simulink model "mcb_pmsm_foc_hall_hvkit_f28069m"  (R2021b)
settings: Solver=FixedStepDiscrete  StartTime=0.0  StopTime=8  RelTol=1e-3  EnableMultiTasking=on
InitFcn:
  | mcb_pmsm_foc_hall_hvkit_f28069m_data;
values from neighbouring files (symbols this model uses):
  inverter = mcb_SetInverterParameters('BoostXL-DRV8305')    [mcb_pmsm_foc_dual_f28379d_data.m]    (also in mcb_pmsm_foc_dual_f28379d_datascript.m; mcb_pmsm_foc_f280049C_data.m; mcb_pmsm_foc_f28335_data.m = mcb_SetInverterParameters('DRV8312-C2-KIT'); mcb_pmsm_foc_hall_f28035_data.m = mcb_SetInverterParameters('DRV8312-C2-KIT'))
  PI_params = mcb.internal.SetControllerParameters(pmsm,inverter,PU_System,T_pwm,2*Ts,Ts_speed)    [mcb_pmsm_foc_dual_f28379d_data.m]    (also in mcb_pmsm_foc_dual_f28379d_datascript.m; mcb_pmsm_foc_f280049C_data.m = mcb.internal.SetControllerParameters(pmsm,inverter,PU_System; mcb_pmsm_foc_f28335_data.m = mcb.internal.SetControllerParameters(pmsm,inverter,PU_System; mcb_pmsm_foc_hall_f28035_data.m = mcb.internal.SetControllerParameters(pmsm,inverter,PU_System)
  pmsm = struct    [c28335_pmsmfoc_data.m]    (also in mcb_pmsm_foc_dual_f28379d_data.m = mcb_SetPMSMMotorParameters('Teknic2310P'); mcb_pmsm_foc_dual_f28379d_datascript.m = mcb_SetPMSMMotorParameters('Teknic2310P'); mcb_pmsm_foc_f280049C_data.m = mcb_SetPMSMMotorParameters('BLY171D'); mcb_pmsm_foc_f28335_data.m = mcb_SetPMSMMotorParameters('BLY171D'))
  target = mcb_SetProcessorDetails('F28379D',PWM_frequency)    [mcb_pmsm_foc_dual_f28379d_data.m]    (also in mcb_pmsm_foc_dual_f28379d_datascript.m; mcb_pmsm_foc_f280049C_data.m = mcb_SetProcessorDetails('F280049C',PWM_frequency); mcb_pmsm_foc_f28335_data.m = mcb_SetProcessorDetails('F28335',PWM_frequency); mcb_pmsm_foc_hall_f28035_data.m = mcb_SetProcessorDetails('F28035',PWM_frequency))
  Ts = 5e-8    (= 5e-08)    [DCDC_Buck_Param.m]    (also in mcb_c2000_open_loop_control_data.m = T_pwm; mcb_c2000_pmsm_offset_data.m = T_pwm; mcb_pmsm_foc_dual_f28379d_data.m = 5e-05; mcb_pmsm_foc_dual_f28379d_datascript.m = 5e-05)
  Ts_motor = T_pwm/2    (= 2.5e-05)    [mcb_pmsm_foc_dual_f28379d_data.m]    (also in mcb_pmsm_foc_dual_f28379d_datascript.m; mcb_pmsm_foc_f280049C_data.m; mcb_pmsm_foc_f28335_data.m; mcb_pmsm_foc_hall_f28035_data.m)
  Ts_simulink = T_pwm/2    (= 2.5e-05)    [mcb_pmsm_foc_dual_f28379d_data.m]    (also in mcb_pmsm_foc_dual_f28379d_datascript.m; mcb_pmsm_foc_f280049C_data.m; mcb_pmsm_foc_f28335_data.m; mcb_pmsm_foc_hall_f28035_data.m)
undefined symbols (not defined in the file or in its folder): Down, GPTRIP1SEL, GPTRIP2SEL, TZ1, TZ2, Up
libraries: simulink x10, mcbpositiondecoderlib x7, idelinklib_common x5, c2802xlib x5, c280xlib x3, c2806xlib x3, svdutilitieslib x2, mcbcontrolslib x2, demo_controls x1, hall_sensor_lib x1, c2000lib x1, mcbplantlib x1
(part 1 of 2)
settings Model: ExtModeTrigDuration=8  Creator=The MathWorks, Inc.  LastModifiedBy=The MathWorks, Inc.
settings SolverCC: AlgebraicLoopSolver=TrustRegion
settings OptimizationCC: DefaultParameterBehavior=Inlined  DefaultUnderspecifiedDataType=single  OptimizeBlockIOStorage=off  EnhancedBackFolding=on  InitFltsAndDblsToZero=on  NoFixptDivByZeroProtection=on  EfficientFloat2IntCast=on  EfficientMapNaN2IntZero=off  MaxStackSize=1024  OptimizeBlockOrder=speed  DifferentSizesBufferReuse=on  DenormalBehavior=FlushToZero  EfficientTunableParamExpr=on
settings DebuggingCC: ReadBeforeWriteMsg=DisableAll  WriteAfterWriteMsg=DisableAll  WriteAfterReadMsg=DisableAll  InheritedTsInSrcMsg=none  MultiTaskDSMMsg=none  TasksWithSamePriorityMsg=none  IntegerOverflowMsg=none  ParameterPrecisionLossMsg=none  ParameterTunabilityLossMsg=error  SFMachineParentedDataDiag=warning  IntegerSaturationMsg=none
settings HardwareCC: ProdBitPerChar=16  ProdBitPerInt=16  ProdBitPerPointer=32  ProdBitPerSizeT=32  ProdBitPerPtrDiffT=32  ProdLargestAtomicInteger=Integer  ProdLargestAtomicFloat=None  ProdWordSize=16  ProdLongLongMode=on  ProdHWDeviceType=Texas Instruments->C2000
settings SFSimCC: MATLABDynamicMemAlloc=off
settings RTWCC: Description=Embedded Coder  SystemTargetFile=ert.tlc  HardwareBoard=TI Piccolo F2806x  TemplateMakefile=ert_default_tmf  GenerateReport=on  Toolchain=Texas Instruments Code Composer Studio (C2000)
settings CodeAppCC: IgnoreCustomStorageClasses=off  StateflowObjectComments=on
settings ERTTargetCC: CodeReplacementLibrary=TI C28x  ExtModeTransport=3  ExtModeStaticAllocSize=2000  ConvertIfToSwitch=off  SuppressUnreachableDefaultCases=off  MemSecPackage=tic2000demospkg

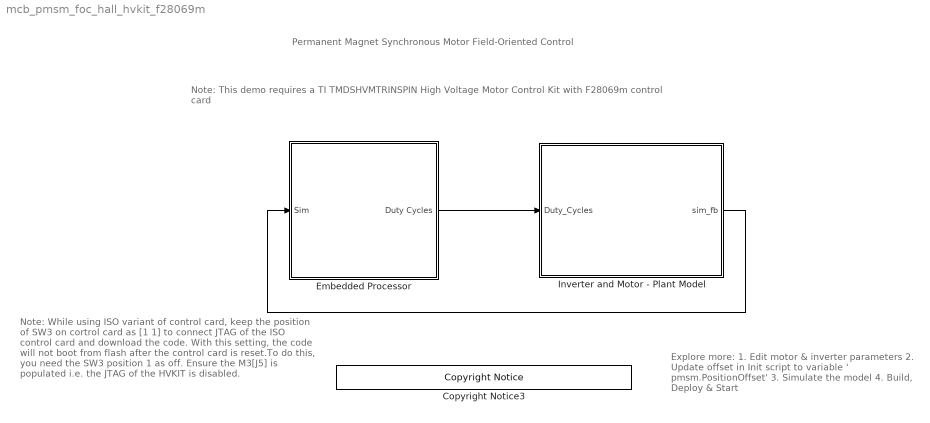
== system mcb_pmsm_foc_hall_hvkit_f28069m ==
  note: Explore more:
      | 1. Edit motor & inverter parameters
      | 2. Update offset in Init script to variable ' pmsm.PositionOffset'
      | 3. Simulate the model
      | 4. Build, Deploy & Start
  note: Permanent Magnet Synchronous Motor Field-Oriented Control
  note: Note: This demo requires a TI TMDSHVMTRINSPIN High Voltage Motor Control Kit with F28069m control card
  note: Note:
      | While using ISO variant of control card, keep the position of SW3 on cortrol card as [1 1] to connect JTAG of the ISO control card and download the code.
      | With this setting, the code will not boot from flash after the control card is reset.To do this, you need the SW3 position 1 as off.
      | Ensure the M3[J5] is populated i.e. the JTAG of the HVKIT is disabled.
  Copyright Notice3 : demo_controls/Copyright Notice  year=2021  prod=tic2000
      settings: SourceProductBaseCode=ME
  Embedded Processor : Subsystem
      mask Display: image('mcb_pmsmfoc_processor.png')
  Inverter and Motor - Plant Model : Subsystem
      mask Display: image('mcb_pmsmfoc_motor.png')
  wires:
  Inverter and Motor - Plant Model/1(sim_fb) -> Embedded Processor/1(Sim)
  Embedded Processor/1(Duty Cycles) -> Inverter and Motor - Plant Model/1(Duty_Cycles)

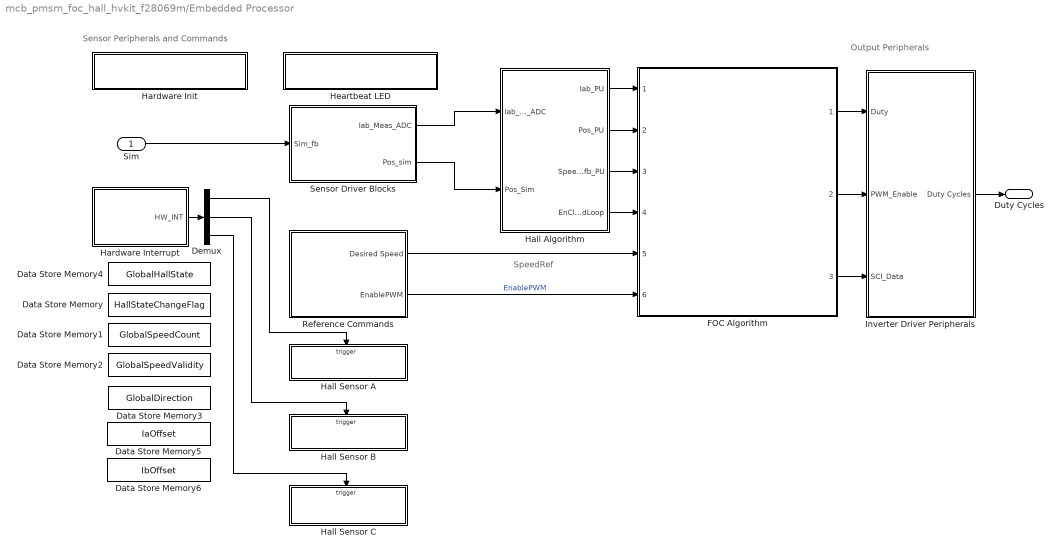
== system mcb_pmsm_foc_hall_hvkit_f28069m/Embedded Processor ==
  note: SpeedRef
  note: Output Peripherals
  note: Sensor Peripherals and Commands
  Sim : Inport
  Data Store Memory : DataStoreMemory  DataStoreName=HallStateChangeFlag  ShowAdditionalParam=off
  Data Store Memory1 : DataStoreMemory  DataStoreName=GlobalSpeedCount  ShowAdditionalParam=off
  Data Store Memory2 : DataStoreMemory  DataStoreName=GlobalSpeedValidity  ShowAdditionalParam=off
  Data Store Memory3 : DataStoreMemory  DataStoreName=GlobalDirection  InitialValue=1  ShowAdditionalParam=off
  Data Store Memory4 : DataStoreMemory  DataStoreName=GlobalHallState  ShowAdditionalParam=off  OutDataTypeStr=uint32
  Data Store Memory5 : DataStoreMemory  DataStoreName=IaOffset  InitialValue=inverter.CtSensAOffset  ShowAdditionalParam=off
  Data Store Memory6 : DataStoreMemory  DataStoreName=IbOffset  InitialValue=inverter.CtSensBOffset  ShowAdditionalParam=off
  Demux : Demux  Outputs=3
  FOC Algorithm : Subsystem  ReferencedSubsystem=foc_hall_algorithm
  Hall Algorithm : Subsystem  TreatAsAtomicUnit=on
      settings: RTWSystemCode=Nonreusable function
  Hall Sensor A : Subsystem
  Hall Sensor B : Subsystem
  Hall Sensor C : Subsystem
  Hardware Init : Subsystem  TreatAsAtomicUnit=on
  Hardware Interrupt : Subsystem  Variant=on  VariantControlMode=sim codegen switching  VariantControl=Choice
  Heartbeat LED : Subsystem  TreatAsAtomicUnit=on
  Inverter Driver Peripherals : Subsystem  TreatAsAtomicUnit=on
      settings: RTWSystemCode=Nonreusable function
  Reference Commands : Subsystem  SystemSampleTime=1e-3
  Sensor Driver Blocks : Subsystem  Variant=on  VariantControlMode=sim codegen switching
  Duty Cycles : Outport
  wires:
  FOC Algorithm/2 -> Inverter Driver Peripherals/2(PWM_Enable)
  Sim/1 -> Sensor Driver Blocks/1(Sim_fb)
  Reference Commands/1(Desired Speed) -> FOC Algorithm/5
  FOC Algorithm/1 -> Inverter Driver Peripherals/1(Duty)
  Inverter Driver Peripherals/1(Duty Cycles) -> Duty Cycles/1
  Reference Commands/2(EnablePWM) -> FOC Algorithm/6  "EnablePWM"
  FOC Algorithm/3 -> Inverter Driver Peripherals/3(SCI_Data)
  Hardware Interrupt/1(HW_INT) -> Demux/1
  Sensor Driver Blocks/1(Iab_Meas_ADC) -> Hall Algorithm/1(Iab_meas_ADC)
  Sensor Driver Blocks/2(Pos_sim) -> Hall Algorithm/2(Pos_Sim)
  Hall Algorithm/1(Iab_PU) -> FOC Algorithm/1
  Hall Algorithm/2(Pos_PU) -> FOC Algorithm/2
  Hall Algorithm/3(Speed_fb_PU) -> FOC Algorithm/3
  Hall Algorithm/4(EnClosedLoop) -> FOC Algorithm/4
  Demux/1 -> Hall Sensor A/Trigger
  Demux/2 -> Hall Sensor B/Trigger
  Demux/3 -> Hall Sensor C/Trigger

== system mcb_pmsm_foc_hall_hvkit_f28069m/Inverter and Motor - Plant Model ==
  Duty_Cycles : Inport
  Bus Creator : BusCreator  Inputs=2
  Plant Model : Subsystem  Variant=on  VariantControlMode=sim codegen switching  VariantControl=Choice
  RT3 : RateTransition  Deterministic=off
  RT4 : RateTransition  Deterministic=off  OutPortSampleTime=Ts
  sim_fb : Outport  VectorParamsAs1DForOutWhenUnconnected=off
  wires:
  Duty_Cycles/1 -> RT3/1
  RT3/1 -> Plant Model/1(Duty_Cycles)
  Plant Model/1(Iab_sim) -> Bus Creator/1  "Iab_sim"
  Plant Model/2(pos_Sim) -> Bus Creator/2  "pos_sim"
  Bus Creator/1 -> RT4/1
  RT4/1 -> sim_fb/1

== system mcb_pmsm_foc_hall_hvkit_f28069m/Embedded Processor/Hall Algorithm ==
  Iab_meas_ADC : Inport
  Pos_Sim : Inport  Port=2
  Input Scaling : Subsystem  Variant=on  VariantControlMode=sim codegen switching  VariantControl=Variant1  PropagateVariantConditions=on
  Iab_PU : Outport
  Pos_PU : Outport  Port=2
  Speed_fb_PU : Outport  Port=3
  EnClosedLoop : Outport  Port=4
  wires:
  Input Scaling/3(Speed_PU) -> Speed_fb_PU/1  "Speed_fb_PU"
  Iab_meas_ADC/1 -> Input Scaling/1(Iab_meas_ADC)
  Input Scaling/4(EnClosedLoop) -> EnClosedLoop/1
  Input Scaling/2(Pos_PU) -> Pos_PU/1  "Pos_PU"
  Pos_Sim/1 -> Input Scaling/2(Pos_Sim)
  Input Scaling/1(Iab_Meas_PU) -> Iab_PU/1  "Iab_PU"

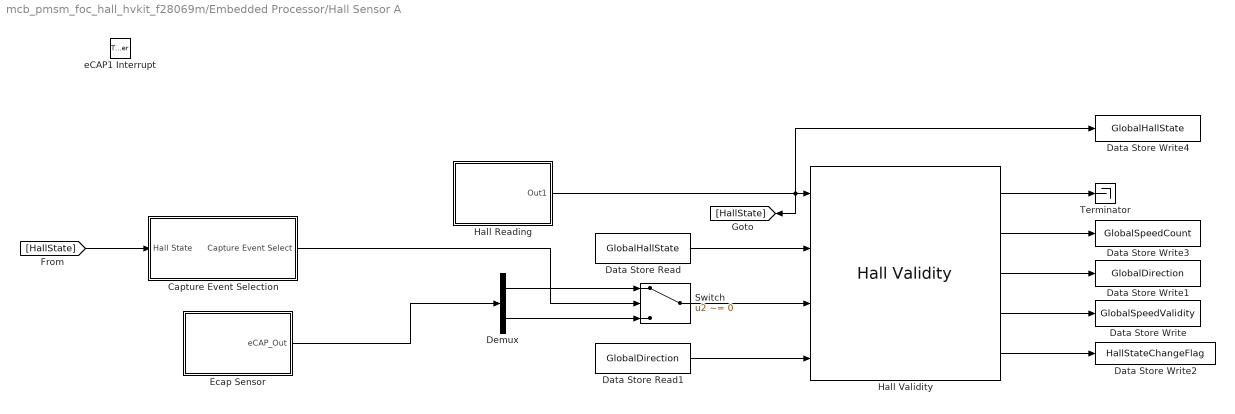
== system mcb_pmsm_foc_hall_hvkit_f28069m/Embedded Processor/Hall Sensor A ==
  eCAP1 Interrupt : TriggerPort  TriggerType=function-call  VariantControl=Variant
  Capture Event Selection : Subsystem
  Data Store Read : DataStoreRead  Priority=1  DataStoreName=GlobalHallState  IndexOptions=Index vector (dialog)  Indices=1  OutputSizes=1
  Data Store Read1 : DataStoreRead  DataStoreName=GlobalDirection  IndexOptions=Index vector (dialog)  Indices=1  OutputSizes=1
  Data Store Write : DataStoreWrite  DataStoreName=GlobalSpeedValidity  IndexOptions=Index vector (dialog)  Indices=1  OutputSizes=1
  Data Store Write1 : DataStoreWrite  DataStoreName=GlobalDirection  IndexOptions=Index vector (dialog)  Indices=1  OutputSizes=1
  Data Store Write2 : DataStoreWrite  DataStoreName=HallStateChangeFlag  IndexOptions=Index vector (dialog)  Indices=1  OutputSizes=1
  Data Store Write3 : DataStoreWrite  DataStoreName=GlobalSpeedCount  IndexOptions=Index vector (dialog)  Indices=1  OutputSizes=1
  Data Store Write4 : DataStoreWrite  Priority=2  DataStoreName=GlobalHallState  IndexOptions=Index vector (dialog)  Indices=1  OutputSizes=1
  Demux : Demux  Outputs=2
  Ecap Sensor : Subsystem  Variant=on  VariantControlMode=sim codegen switching  VariantControl=Choice
  Hall Reading : Subsystem  Variant=on  VariantControlMode=sim codegen switching  VariantControl=Choice
  Hall Validity : mcbpositiondecoderlib/Hall Validity  hallSequence=ABC  sequence=[5,4,6,2,3,1]  CounterSize=32 bits
      settings: SourceProductBaseCode=MT
  Switch : Switch  Criteria=u2 ~= 0
  Terminator : Terminator
  wires:
  Hall Validity/3 -> Data Store Write1/1
  Hall Validity/5 -> Data Store Write2/1
  Hall Validity/4 -> Data Store Write/1
  Data Store Read/1 -> Hall Validity/2
  Data Store Read1/1 -> Hall Validity/4
  Switch/1 -> Hall Validity/3
  Hall Validity/2 -> Data Store Write3/1
  Demux/2 -> Switch/3
  Demux/1 -> Switch/1
  Hall Validity/1 -> Terminator/1
  [HallState] -> Capture Event Selection/1(Hall State)
  Ecap Sensor/1(eCAP_Out) -> Demux/1
  Hall Reading/1(Out1) -> Data Store Write4/1, [HallState], Hall Validity/1
  Capture Event Selection/1(Capture Event Select) -> Switch/2

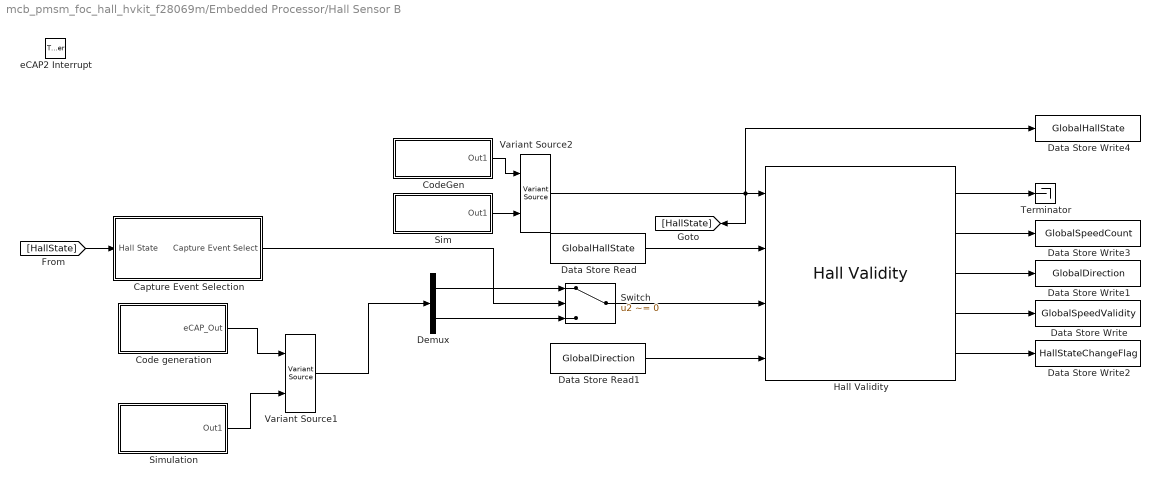
== system mcb_pmsm_foc_hall_hvkit_f28069m/Embedded Processor/Hall Sensor B ==
  eCAP2 Interrupt : TriggerPort  TriggerType=function-call  VariantControl=Variant
  Capture Event Selection : Subsystem
  Code generation : Subsystem
  CodeGen : Subsystem
  Data Store Read : DataStoreRead  Priority=1  DataStoreName=GlobalHallState  IndexOptions=Index vector (dialog)  Indices=1  OutputSizes=1
  Data Store Read1 : DataStoreRead  DataStoreName=GlobalDirection  IndexOptions=Index vector (dialog)  Indices=1  OutputSizes=1
  Data Store Write : DataStoreWrite  DataStoreName=GlobalSpeedValidity  IndexOptions=Index vector (dialog)  Indices=1  OutputSizes=1
  Data Store Write1 : DataStoreWrite  DataStoreName=GlobalDirection  IndexOptions=Index vector (dialog)  Indices=1  OutputSizes=1
  Data Store Write2 : DataStoreWrite  DataStoreName=HallStateChangeFlag  IndexOptions=Index vector (dialog)  Indices=1  OutputSizes=1
  Data Store Write3 : DataStoreWrite  DataStoreName=GlobalSpeedCount  IndexOptions=Index vector (dialog)  Indices=1  OutputSizes=1
  Data Store Write4 : DataStoreWrite  Priority=2  DataStoreName=GlobalHallState  IndexOptions=Index vector (dialog)  Indices=1  OutputSizes=1
  Demux : Demux  Outputs=2
  Hall Validity : mcbpositiondecoderlib/Hall Validity  hallSequence=ABC  sequence=[5,4,6,2,3,1]  CounterSize=32 bits
      settings: SourceProductBaseCode=MT
  Sim : Subsystem
  Simulation : Subsystem
  Switch : Switch  Criteria=u2 ~= 0  Threshold=3
  Terminator : Terminator
  Variant Source1 : VariantSource  VariantControlMode=sim codegen switching
  Variant Source2 : VariantSource  VariantControlMode=sim codegen switching
  wires:
  Hall Validity/3 -> Data Store Write1/1
  Hall Validity/5 -> Data Store Write2/1
  Hall Validity/4 -> Data Store Write/1
  Data Store Read1/1 -> Hall Validity/4
  Hall Validity/2 -> Data Store Write3/1
  Data Store Read/1 -> Hall Validity/2
  Demux/1 -> Switch/1
  Demux/2 -> Switch/3
  Variant Source1/1 -> Demux/1
  Switch/1 -> Hall Validity/3
  Hall Validity/1 -> Terminator/1
  [HallState] -> Capture Event Selection/1(Hall State)
  Capture Event Selection/1(Capture Event Select) -> Switch/2
  Code generation/1(eCAP_Out) -> Variant Source1/1
  Simulation/1(Out1) -> Variant Source1/2
  Variant Source2/1 -> Data Store Write4/1, Hall Validity/1, [HallState]
  CodeGen/1(Out1) -> Variant Source2/1
  Sim/1(Out1) -> Variant Source2/2

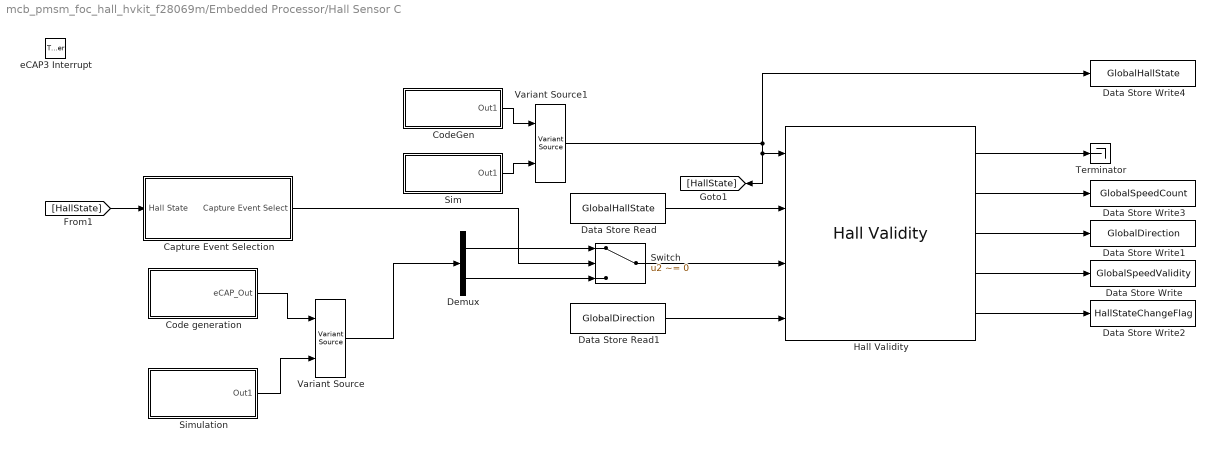
== system mcb_pmsm_foc_hall_hvkit_f28069m/Embedded Processor/Hall Sensor C ==
  eCAP3 Interrupt : TriggerPort  TriggerType=function-call  VariantControl=Variant
  Capture Event Selection : Subsystem
  Code generation : Subsystem
  CodeGen : Subsystem
  Data Store Read : DataStoreRead  Priority=1  DataStoreName=GlobalHallState  IndexOptions=Index vector (dialog)  Indices=1  OutputSizes=1
  Data Store Read1 : DataStoreRead  DataStoreName=GlobalDirection  IndexOptions=Index vector (dialog)  Indices=1  OutputSizes=1
  Data Store Write : DataStoreWrite  DataStoreName=GlobalSpeedValidity  IndexOptions=Index vector (dialog)  Indices=1  OutputSizes=1
  Data Store Write1 : DataStoreWrite  DataStoreName=GlobalDirection  IndexOptions=Index vector (dialog)  Indices=1  OutputSizes=1
  Data Store Write2 : DataStoreWrite  DataStoreName=HallStateChangeFlag  IndexOptions=Index vector (dialog)  Indices=1  OutputSizes=1
  Data Store Write3 : DataStoreWrite  DataStoreName=GlobalSpeedCount  IndexOptions=Index vector (dialog)  Indices=1  OutputSizes=1
  Data Store Write4 : DataStoreWrite  Priority=2  DataStoreName=GlobalHallState  IndexOptions=Index vector (dialog)  Indices=1  OutputSizes=1
  Demux : Demux  Outputs=2
  Hall Validity : mcbpositiondecoderlib/Hall Validity  hallSequence=ABC  sequence=[5,4,6,2,3,1]  CounterSize=32 bits
      settings: SourceProductBaseCode=MT
  Sim : Subsystem
  Simulation : Subsystem
  Switch : Switch  Criteria=u2 ~= 0  Threshold=3
  Terminator : Terminator
  Variant Source : VariantSource  VariantControlMode=sim codegen switching
  Variant Source1 : VariantSource  VariantControlMode=sim codegen switching
  wires:
  Hall Validity/3 -> Data Store Write1/1
  Hall Validity/5 -> Data Store Write2/1
  Hall Validity/4 -> Data Store Write/1
  Data Store Read1/1 -> Hall Validity/4
  Hall Validity/2 -> Data Store Write3/1
  Data Store Read/1 -> Hall Validity/2
  Demux/1 -> Switch/1
  Demux/2 -> Switch/3
  Variant Source/1 -> Demux/1
  Switch/1 -> Hall Validity/3
  Hall Validity/1 -> Terminator/1
  [HallState] -> Capture Event Selection/1(Hall State)
  Capture Event Selection/1(Capture Event Select) -> Switch/2
  Code generation/1(eCAP_Out) -> Variant Source/1
  Simulation/1(Out1) -> Variant Source/2
  Variant Source1/1 -> [HallState], Hall Validity/1, Data Store Write4/1
  CodeGen/1(Out1) -> Variant Source1/1
  Sim/1(Out1) -> Variant Source1/2

== system mcb_pmsm_foc_hall_hvkit_f28069m/Embedded Processor/Hardware Init ==
  Event Listener : EventListener  DisableCoverage=on  EventName=reset
  Offset Calculation : Subsystem  Variant=on  VariantControlMode=sim codegen switching  VariantControl=Choice

== system mcb_pmsm_foc_hall_hvkit_f28069m/Embedded Processor/Hardware Interrupt ==
  Code Generation : Subsystem  VariantControl=(codegen)
  Simulation : Subsystem  VariantControl=(sim)
  HW_INT : Outport  OutputFunctionCall=on

== system mcb_pmsm_foc_hall_hvkit_f28069m/Embedded Processor/Heartbeat LED ==
  note: Heartbeat LED 1HZ
  LED BLINK : Subsystem  Variant=on  VariantControlMode=sim codegen switching  VariantControl=Choice
  RED_LED : Constant  OutDataTypeStr=uint16  SampleTime=0.5
  wires:
  RED_LED/1 -> LED BLINK/1(In1)

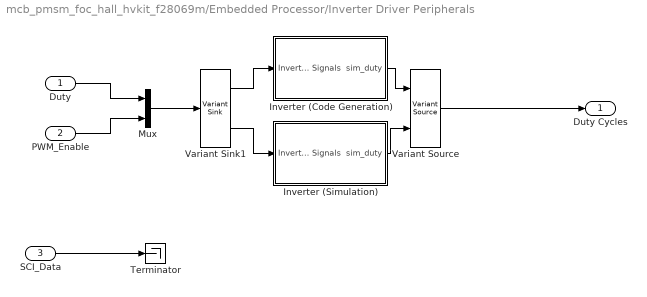
== system mcb_pmsm_foc_hall_hvkit_f28069m/Embedded Processor/Inverter Driver Peripherals ==
  Duty : Inport
  PWM_Enable : Inport  Port=2
  SCI_Data : Inport  Port=3
  Inverter (Code Generation) : Subsystem  VariantControl=Choice
  Inverter (Simulation) : Subsystem  VariantControl=(sim)
  Mux : Mux  Inputs=2
  Terminator : Terminator
  Variant Sink1 : VariantSink  VariantControlMode=sim codegen switching
  Variant Source : VariantSource  VariantControlMode=sim codegen switching
  Duty Cycles : Outport  InitialOutput=0  VectorParamsAs1DForOutWhenUnconnected=off
  wires:
  Variant Source/1 -> Duty Cycles/1
  PWM_Enable/1 -> Mux/2
  Duty/1 -> Mux/1
  Variant Sink1/2 -> Inverter (Simulation)/1(Inverter Signals)
  Inverter (Code Generation)/1(sim_duty) -> Variant Source/1
  Mux/1 -> Variant Sink1/1
  Variant Sink1/1 -> Inverter (Code Generation)/1(Inverter Signals)
  Inverter (Simulation)/1(sim_duty) -> Variant Source/2
  SCI_Data/1 -> Terminator/1

== system mcb_pmsm_foc_hall_hvkit_f28069m/Embedded Processor/Reference Commands ==
  Data Type Conversion3 : DataTypeConversion  OutDataTypeStr=boolean  RndMeth=Simplest
  Enable PWM : Constant  OutDataTypeStr=uint16
  Speed Command in PU : Constant  Value=0.5  OutDataTypeStr=dataType
  Desired Speed : Outport  VectorParamsAs1DForOutWhenUnconnected=off
  EnablePWM : Outport  Port=2
  wires:
  Data Type Conversion3/1 -> EnablePWM/1
  Speed Command in PU/1 -> Desired Speed/1  "Speed_Ref"
  Enable PWM/1 -> Data Type Conversion3/1

== system mcb_pmsm_foc_hall_hvkit_f28069m/Embedded Processor/Sensor Driver Blocks ==
  Sim_fb : Inport
  Sensor Driver Blocks (codegen) : Subsystem  VariantControl=(codegen)
  Sensor Driver Blocks (sim) : Subsystem  VariantControl=(sim)
  Iab_Meas_ADC : Outport
  Pos_sim : Outport  Port=2

== system mcb_pmsm_foc_hall_hvkit_f28069m/Inverter and Motor - Plant Model/Plant Model ==
  Duty_Cycles : Inport
  Codegeneration : Subsystem  VariantControl=(codegen)
  Simulation : Subsystem  VariantControl=(sim)
  Iab_sim : Outport
  pos_Sim : Outport  Port=2

== system mcb_pmsm_foc_hall_hvkit_f28069m/Embedded Processor/Hall Algorithm/Input Scaling ==
  note: Variant control to pass plant simulated value for simulation and
      | ADC measured value for codegen.
  Iab_meas_ADC : Inport
  Pos_Sim : Inport  Port=2
  Read_Sensor (codegen) : Subsystem  VariantControl=(codegen)
  Read_Sensor (sim) : Subsystem  VariantControl=(sim)
  Iab_Meas_PU : Outport  VectorParamsAs1DForOutWhenUnconnected=off
  Pos_PU : Outport  Port=2  VectorParamsAs1DForOutWhenUnconnected=off
  Speed_PU : Outport  Port=3  VectorParamsAs1DForOutWhenUnconnected=off
  EnClosedLoop : Outport  Port=4  VectorParamsAs1DForOutWhenUnconnected=off

== system mcb_pmsm_foc_hall_hvkit_f28069m/Embedded Processor/Hall Sensor A/Capture Event Selection ==
  Hall State : Inport
  If : If  IfExpression=(u1 == 5 | u1 == 3)
  Merge : Merge
  Output 0 : Subsystem  TreatAsAtomicUnit=on
  Output 1 : Subsystem  TreatAsAtomicUnit=on
  Capture Event Select : Outport
  wires:
  Output 1/1(Out1) -> Merge/2
  Output 0/1(Out1) -> Merge/1
  If/2 -> Output 1/Action
  If/1 -> Output 0/Action
  Hall State/1 -> If/1
  Merge/1 -> Capture Event Select/1

== system mcb_pmsm_foc_hall_hvkit_f28069m/Embedded Processor/Hall Sensor A/Ecap Sensor ==
  Code generation : Subsystem  VariantControl=(codegen)
  Simulation : Subsystem  VariantControl=(sim)
  eCAP_Out : Outport

== system mcb_pmsm_foc_hall_hvkit_f28069m/Embedded Processor/Hall Sensor A/Hall Reading ==
  CodeGen : Subsystem  VariantControl=(codegen)
  Sim : Subsystem  VariantControl=(sim)
  Out1 : Outport

== system mcb_pmsm_foc_hall_hvkit_f28069m/Embedded Processor/Hall Sensor B/Capture Event Selection ==
  Hall State : Inport
  If : If  IfExpression=(u1 == 3 | u1 == 6)
  Merge : Merge
  Output 0 : Subsystem  TreatAsAtomicUnit=on
  Output 1 : Subsystem  TreatAsAtomicUnit=on
  Capture Event Select : Outport
  wires:
  Output 1/1(Out1) -> Merge/1
  Output 0/1(Out1) -> Merge/2
  If/2 -> Output 0/Action
  If/1 -> Output 1/Action
  Hall State/1 -> If/1
  Merge/1 -> Capture Event Select/1

== system mcb_pmsm_foc_hall_hvkit_f28069m/Embedded Processor/Hall Sensor B/Code generation ==
  eCAP : c280xlib/eCAP  operatingMode=eCAP  selectCAPx=eCAP2  offsetValue=0  counterSynIn=off  enableCounter=off  syncOutput=Disabled  sampleTime=-1  eventPrescaler=0  selectMode=Continuous  enableOneShot=off  stopValue=Capture Event 2  resetEv1Ts=on  ev1Polarity=Rising Edge  resetEv2Ts=on  ev2Polarity=Falling Edge  resetEv3Ts=off  ev3Polarity=Rising Edge  resetEv4Ts=off  ev4Polarity=Rising Edge  tSCntrDataType=uint32  capEvFlag=off  capFlagDataType=uint16  overFlowFlag=off  overFlowFlagDataType=uint16  periodUnit=Seconds  periodSource=Specify via dialog  waveformPeriod=0.001  dutyUnit=Percentages  dutySource=Specify via dialog  dutyCycle=50  outputPolarity=Active High  enableCEVT1Int=on  enableCEVT2Int=on  enableCEVT3Int=off  enableCEVT4Int=off  enableCTROVFInt=on  enablePRDInt=off  enableCMPInt=off
      settings: SourceProductBaseCode=TIC2000
  eCAP_Out : Outport
  wires:
  eCAP/1 -> eCAP_Out/1

== system mcb_pmsm_foc_hall_hvkit_f28069m/Embedded Processor/Hall Sensor B/CodeGen ==
  Bitwise AND : simulink/Logic and Bit Operations/Bitwise Operator  logicop=AND  UseBitMask=on  BitMask=hex2dec('07000000')  BitMaskRealWorld=Stored Integer
  Data Type Conversion : DataTypeConversion  OutDataTypeStr=uint32  ConvertRealWorld=Stored Integer (SI)
  Memory Copy : idelinklib_common/Memory Copy  copyFrom=Specified source code symbol  copyFromAddressSource=Specify via dialog  copyFromAddress=hex2dec('00001000')  copyFromSrcCode=&GpioDataRegs.GPADAT.all  dataTypeFrom=uint32  dataDimensionFrom=1  useOffsetFrom=off  offsetFromSrc=Specify via dialog  offsetFrom=0  strideFrom=1  copyTo=Output port  copyToAddressSource=Specify via dialog  copyToAddress=hex2dec('00002000')  copyToSrcCode=myVariableDst  dataTypeTo=uint32  useOffsetTo=off  offsetToSrc=Specify via dialog  offsetTo=0  strideTo=1  sampleTime=-1  useInitValue=off  initValueSrc=Specify constant value  initValue=1  initValueSrcCode=myInitValueVariable  useAsMask=off  maskOperator=bitwise AND  useTermValue=off  termValue=1  isRealtimeEnabled=off  emitCCBeforeWrite=off  CCBeforeWrite=/* Custom Code Before Write*/  emitCCAfterWrite=off  CCAfterWrite=/* Custom Code After Write*/  useDMACopy=off  enableBlockingMode=off
      settings: SourceProductBaseCode=ME
  Shift Arithmetic : ArithShift  BitShiftNumber=24
  Out1 : Outport
  wires:
  Memory Copy/1 -> Bitwise AND/1
  Data Type Conversion/1 -> Out1/1
  Bitwise AND/1 -> Shift Arithmetic/1
  Shift Arithmetic/1 -> Data Type Conversion/1

== system mcb_pmsm_foc_hall_hvkit_f28069m/Embedded Processor/Hall Sensor B/Sim ==
  Data Type Conversion : DataTypeConversion  OutDataTypeStr=uint32  ConvertRealWorld=Stored Integer (SI)
  Ground : Ground
  Out1 : Outport
  wires:
  Data Type Conversion/1 -> Out1/1
  Ground/1 -> Data Type Conversion/1

== system mcb_pmsm_foc_hall_hvkit_f28069m/Embedded Processor/Hall Sensor B/Simulation ==
  Ground : Ground
  Ground1 : Ground
  Mux : Mux  Inputs=2
  Out1 : Outport
  wires:
  Ground1/1 -> Mux/2
  Mux/1 -> Out1/1
  Ground/1 -> Mux/1

== system mcb_pmsm_foc_hall_hvkit_f28069m/Embedded Processor/Hall Sensor C/Capture Event Selection ==
  Hall State : Inport
  If : If  IfExpression=(u1 == 5 | u1 == 6)
  Merge : Merge
  Output 0 : Subsystem  TreatAsAtomicUnit=on
  Output 1 : Subsystem  TreatAsAtomicUnit=on
  Capture Event Select : Outport
  wires:
  Output 1/1(Out1) -> Merge/1
  Output 0/1(Out1) -> Merge/2
  If/2 -> Output 0/Action
  If/1 -> Output 1/Action
  Hall State/1 -> If/1
  Merge/1 -> Capture Event Select/1

== system mcb_pmsm_foc_hall_hvkit_f28069m/Embedded Processor/Hall Sensor C/Code generation ==
  eCAP : c280xlib/eCAP  operatingMode=eCAP  selectCAPx=eCAP3  offsetValue=0  counterSynIn=off  enableCounter=off  syncOutput=Disabled  sampleTime=-1  eventPrescaler=0  selectMode=Continuous  enableOneShot=off  stopValue=Capture Event 2  resetEv1Ts=on  ev1Polarity=Rising Edge  resetEv2Ts=on  ev2Polarity=Falling Edge  resetEv3Ts=off  ev3Polarity=Rising Edge  resetEv4Ts=off  ev4Polarity=Rising Edge  tSCntrDataType=uint32  capEvFlag=off  capFlagDataType=uint16  overFlowFlag=off  overFlowFlagDataType=uint16  periodUnit=Seconds  periodSource=Specify via dialog  waveformPeriod=0.001  dutyUnit=Percentages  dutySource=Specify via dialog  dutyCycle=50  outputPolarity=Active High  enableCEVT1Int=on  enableCEVT2Int=on  enableCEVT3Int=off  enableCEVT4Int=off  enableCTROVFInt=on  enablePRDInt=off  enableCMPInt=off
      settings: SourceProductBaseCode=TIC2000
  eCAP_Out : Outport
  wires:
  eCAP/1 -> eCAP_Out/1

== system mcb_pmsm_foc_hall_hvkit_f28069m/Embedded Processor/Hall Sensor C/CodeGen ==
  Bitwise AND : simulink/Logic and Bit Operations/Bitwise Operator  logicop=AND  UseBitMask=on  BitMask=hex2dec('07000000')  BitMaskRealWorld=Stored Integer
  Data Type Conversion : DataTypeConversion  OutDataTypeStr=uint32  ConvertRealWorld=Stored Integer (SI)
  Memory Copy : idelinklib_common/Memory Copy  copyFrom=Specified source code symbol  copyFromAddressSource=Specify via dialog  copyFromAddress=hex2dec('00001000')  copyFromSrcCode=&GpioDataRegs.GPADAT.all  dataTypeFrom=uint32  dataDimensionFrom=1  useOffsetFrom=off  offsetFromSrc=Specify via dialog  offsetFrom=0  strideFrom=1  copyTo=Output port  copyToAddressSource=Specify via dialog  copyToAddress=hex2dec('00002000')  copyToSrcCode=myVariableDst  dataTypeTo=uint32  useOffsetTo=off  offsetToSrc=Specify via dialog  offsetTo=0  strideTo=1  sampleTime=-1  useInitValue=off  initValueSrc=Specify constant value  initValue=1  initValueSrcCode=myInitValueVariable  useAsMask=off  maskOperator=bitwise AND  useTermValue=off  termValue=1  isRealtimeEnabled=off  emitCCBeforeWrite=off  CCBeforeWrite=/* Custom Code Before Write*/  emitCCAfterWrite=off  CCAfterWrite=/* Custom Code After Write*/  useDMACopy=off  enableBlockingMode=off
      settings: SourceProductBaseCode=ME
  Shift Arithmetic : ArithShift  BitShiftNumber=24
  Out1 : Outport
  wires:
  Data Type Conversion/1 -> Out1/1
  Shift Arithmetic/1 -> Data Type Conversion/1
  Bitwise AND/1 -> Shift Arithmetic/1
  Memory Copy/1 -> Bitwise AND/1

== system mcb_pmsm_foc_hall_hvkit_f28069m/Embedded Processor/Hall Sensor C/Sim ==
  Data Type Conversion : DataTypeConversion  OutDataTypeStr=uint32  ConvertRealWorld=Stored Integer (SI)
  Ground : Ground
  Out1 : Outport
  wires:
  Data Type Conversion/1 -> Out1/1
  Ground/1 -> Data Type Conversion/1

== system mcb_pmsm_foc_hall_hvkit_f28069m/Embedded Processor/Hall Sensor C/Simulation ==
  Ground : Ground
  Ground1 : Ground
  Mux : Mux  Inputs=2
  Out1 : Outport
  wires:
  Ground1/1 -> Mux/2
  Mux/1 -> Out1/1
  Ground/1 -> Mux/1

== system mcb_pmsm_foc_hall_hvkit_f28069m/Embedded Processor/Hardware Init/Offset Calculation ==
  Code Generation : Subsystem  VariantControl=(codegen)
  Simulation : Subsystem  VariantControl=(sim)

== system mcb_pmsm_foc_hall_hvkit_f28069m/Embedded Processor/Hardware Interrupt/Code Generation ==
  Hardware Interrupt : c2000lib/Scheduling/C28x Hardware Interrupt  irqnumbers=[4 4 4]  pienumbers=[1 2 3]  irqpriorities=[25 25 25]  irqpreempts=[0 0 0]  showinput=off  dspchiptype=C280X
      settings: SourceProductBaseCode=TIC2000
  HW_INT : Outport  VectorParamsAs1DForOutWhenUnconnected=off
  wires:
  Hardware Interrupt/1 -> HW_INT/1

== system mcb_pmsm_foc_hall_hvkit_f28069m/Embedded Processor/Hardware Interrupt/Simulation ==
  Function-Call Generator1 : simulink/Ports & Subsystems/Function-Call Generator  sample_time=Ts  numberOfIterations=1  DisallowWideOutput=off
  Function-Call Generator3 : simulink/Ports & Subsystems/Function-Call Generator  sample_time=Ts  numberOfIterations=1  DisallowWideOutput=off
  Function-Call Generator4 : simulink/Ports & Subsystems/Function-Call Generator  sample_time=Ts  numberOfIterations=1  DisallowWideOutput=off
  Mux : Mux  Inputs=3
  HW_INT : Outport  VectorParamsAs1DForOutWhenUnconnected=off
  wires:
  Mux/1 -> HW_INT/1
  Function-Call Generator1/1 -> Mux/1
  Function-Call Generator3/1 -> Mux/2
  Function-Call Generator4/1 -> Mux/3

== system mcb_pmsm_foc_hall_hvkit_f28069m/Embedded Processor/Heartbeat LED/LED BLINK ==
  In1 : Inport
  Code generation : Subsystem  VariantControl=(codegen)
  Simulation : Subsystem  VariantControl=(sim)

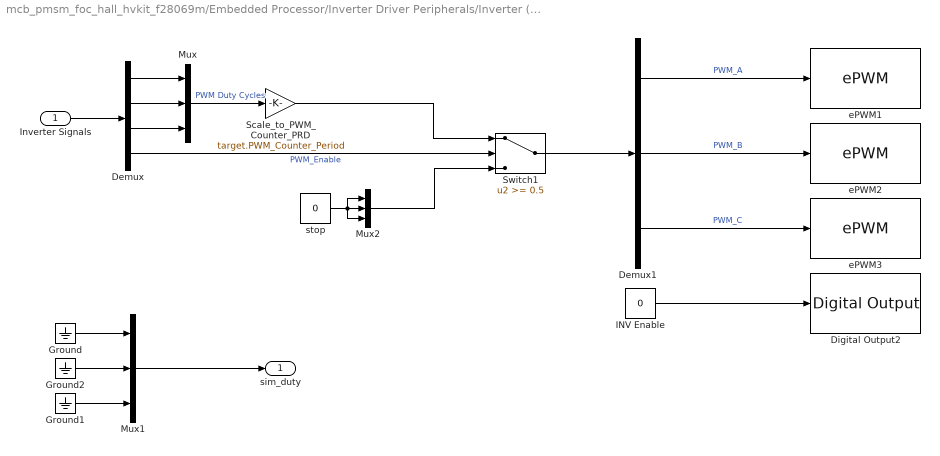
== system mcb_pmsm_foc_hall_hvkit_f28069m/Embedded Processor/Inverter Driver Peripherals/Inverter (Code Generation) ==
  Inverter Signals : Inport
  Demux : Demux
  Demux1 : Demux  Outputs=3
  Digital Output2 : c2806xlib/Digital Output  GPIO_Number=GPIO8~GPIO15  GPIO_Bit0=off  GPIO_BIT0_Toggle=off  GPIO_Bit1=off  GPIO_BIT1_Toggle=off  GPIO_Bit2=off  GPIO_BIT2_Toggle=off  GPIO_Bit3=off  GPIO_BIT3_Toggle=off  GPIO_Bit4=off  GPIO_BIT4_Toggle=off  GPIO_Bit5=off  GPIO_BIT5_Toggle=off  GPIO_Bit6=off  GPIO_BIT6_Toggle=off  GPIO_Bit7=on  GPIO_BIT7_Toggle=off
      settings: SourceProductBaseCode=TIC2000
  Ground : Ground
  Ground1 : Ground
  Ground2 : Ground
  INV Enable : Constant  Value=0  OutDataTypeStr=uint16
  Mux : Mux  Inputs=3
  Mux1 : Mux  Inputs=3
  Mux2 : Mux  Inputs=3
  Scale_to_PWM_Counter_PRD : Gain  Gain=target.PWM_Counter_Period  OutDataTypeStr=uint16  RndMeth=Simplest
  Switch1 : Switch  Threshold=0.5
  ePWM1 : c2802xlib/ePWM  PwmType=C2000  useModule=ePWM1  ePWMxLINKTBPRD=Not Linked  periodUnits=Clock cycles  timerSource=Specify via dialog  timerPeriod_clk=target.PWM_Counter_Period+1  timerPeriod_sec=64000  tbshadow=Counter equals to zero  countingMode=Up-Down  phaseActiveEnable=Disable  phaseDirection=Count down after sync  phaseActive=0  synchronizationEnable=off  dcaevt1Sync=off  dcbevt1Sync=off  synchronizationOption=Counter equals to zero (CTR=Zero)  perSynchronizationOption=Counter equals to period (CTR=PRD)  clockPrescale=1  HSclockPrescale=1  enswap=off  ePWMxAStatus=on  ePWMxAactionLogic1=Do nothing  ePWMxAactionLogic2=Do nothing  ePWMxAactionLogic3=Clear  ePWMxAactionLogic4=Set  ePWMxAactionLogic5=Do nothing  ePWMxAactionLogic6=Do nothing  ePWMxACSFenable=off  ePWMxACSFvalue=Forcing disable  ePWMxASFreload=Zero  ePWMxBStatus=off  ePWMxBactionLogic1=Do nothing  ePWMxBactionLogic2=Set  ePWMxBactionLogic3=Do nothing  ePWMxBactionLogic4=Do nothing  ePWMxBactionLogic5=Clear  ePWMxBactionLogic6=Do nothing  ePWMxBCSFenable=off  ePWMxBCSFvalue=Forcing disable  ePWMxBSFreload=Zero  ePWNxBOutWay=off  ePWMxLINKCMPA=Not Linked  CMPAUnits=Clock cycles  CMPASource=Input port  CMPAValue_per=32000  CMPAValue_clk=target.PWM_Counter_Period/2+1  enCMPAshadow=Counter equals to zero (CTR=Zero)  ePWMxLINKCMPB=Not Linked  CMPBUnits=Clock cycles  CMPBSource=Specify via dialog  CMPBValue_per=50  CMPBValue_clk=target.PWM_Counter_Period/2+1  enCMPBshadow=Counter equals to zero (CTR=Zero)  ePWMxLINKCMPC=Not Linked  CMPCUnits=Clock cycles  CMPCSource=Specify via dialog  CMPCValue_per=50  CMPCValue_clk=32000  enCMPCshadow=Counter equals to zero (CTR=Zero)  ePWMxLINKCMPD=Not Linked  CMPDUnits=Clock cycles  CMPDSource=Specify via dialog  CMPDValue_per=50  CMPDValue_clk=32000  enCMPDshadow=Counter equals to zero (CTR=Zero)  enableDBePWMxA=on  enableDBePWMxB=on  enhalfcycle=off  DBpolarity=Active high complementary (AHC)  DBedgeDelay=Positive  DBSource_ePWMxA=ePWMxA  DBSource_ePWMxB=ePWMxA  DBPeriodUnits=Clock cycles  DBperiodSource=Specify via dialog  REDperiod=15  FEDperiod=15  REDperiod_sec=0  FEDperiod_sec=0  LoadModeDBRED=Immediate without using shadow  LoadModeDBFED=Immediate without using shadow  adcstartModuleA=on  adcrequestEventA=First event  adcstartEventA=Counter equals to period (CTR=PRD)  adcstartEventA_type2=Digital Compare Module A Event 1 start of conversion (DCAEVT1.soc)  adcstartModuleB=off  adcrequestEventB=First event  adcstartEventB=Counter equals to zero (CTR=Zero)  adcstartEventB_type2=Counter equals to zero (CTR=Zero)  intEn=off  intPrd=First event  intSel=Counter equals to zero (CTR=Zero)  intSel_type2=Counter equals to zero (CTR=Zero)  hrpe=off  enHRPWM=off  HRPWM_LoadMode=Counter equals to period (CTR=PRD)  HRPWM_CTLMode=Duty or Period control mode  HRPWM_EDGMode=Both edge  hrpeb=off  enHRPWMB=off  HRPWM_LoadModeB=Counter equals to zero (CTR=ZERO)  HRPWM_CTLModeB=Duty or Period control mode  HRPWM_EDGModeB=Both edge  enHRDBRED=off  enHRDBFED=off  enSFO=on  enautoconv=on  chopperEnable=off  chopperFrequency=1  chopperFirstwidth=1  chopperDuty=12.5%  tripZonesource=Specify via dialog  tzselOSHT1=off  tzselOSHT2=off  tzselOSHT3=off  tzselOSHDCAEV1=off  tzselOSHDCBEV1=off  tzselCBC1=off  tzselCBC2=off  tzselCBC3=off  tzselCBCDCAEV2=off  tzselCBCDCBEV2=off  tzselOSHT4=off  tzselOSHT5=off  tzselOSHT6=off  tzselCBC4=off  tzselCBC5=off  tzselCBC6=off  enTzOstIntr=off  enTzCbcIntr=off  enTzDCAEVT1Intr=off  enTzDCAEVT2Intr=off  enTzDCBEVT1Intr=off  enTzDCBEVT2Intr=off  ePWMxAforced=No action  ePWMxBforced=No action  DCAEVT1forced=No action  DCBEVT1forced=No action  DCAEVT2forced=No action  DCBEVT2forced=No action  dcah=Trip Zone 1 input (TZ1)  dcal=Trip Zone 2 input (TZ2)  dcbh=Trip Zone 1 input (TZ1)  dcbl=Trip Zone 2 input (TZ2)  dcah_type2=GPTRIP1SEL/(TZ1)  dcal_type2=GPTRIP2SEL/(TZ2)  dcbh_type2=GPTRIP1SEL/(TZ1)  dcbl_type2=GPTRIP2SEL/(TZ2)  gendcaevt1=Event disabled  gendcaevt2=Event disabled  gendcbevt1=Event disabled  gendcbevt2=Event disabled  dcaevt1src=DCAEVT1 with sync  dcaevt2src=DCAEVT2 with sync  dcbevt1src=DCBEVT1 with sync  dcbevt2src=DCBEVT2 with sync  pulsesel=Counter equals to zero (CTR=Zero)  blankinv=off  blankoffset=0  blankwidth=0  evsrcsel=Filtered version of DCAEVT1 (DCAEVT1FILT)  encape=off
  ePWM2 : c2802xlib/ePWM  PwmType=C2000  useModule=ePWM2  ePWMxLINKTBPRD=Not Linked  periodUnits=Clock cycles  timerSource=Specify via dialog  timerPeriod_clk=target.PWM_Counter_Period+1  timerPeriod_sec=64000  tbshadow=Counter equals to zero  countingMode=Up-Down  phaseActiveEnable=Set counter to phase value specified via dialog  phaseDirection=Count up after sync  phaseActive=0  synchronizationEnable=off  dcaevt1Sync=off  dcbevt1Sync=off  synchronizationOption=Pass through (EPWMxSYNCI or SWFSYNC)  perSynchronizationOption=Counter equals to period (CTR=PRD)  clockPrescale=1  HSclockPrescale=1  enswap=off  ePWMxAStatus=on  ePWMxAactionLogic1=Do nothing  ePWMxAactionLogic2=Do nothing  ePWMxAactionLogic3=Clear  ePWMxAactionLogic4=Set  ePWMxAactionLogic5=Do nothing  ePWMxAactionLogic6=Do nothing  ePWMxACSFenable=off  ePWMxACSFvalue=Forcing disable  ePWMxASFreload=Zero  ePWMxBStatus=off  ePWMxBactionLogic1=Do nothing  ePWMxBactionLogic2=Set  ePWMxBactionLogic3=Do nothing  ePWMxBactionLogic4=Do nothing  ePWMxBactionLogic5=Clear  ePWMxBactionLogic6=Do nothing  ePWMxBCSFenable=off  ePWMxBCSFvalue=Forcing disable  ePWMxBSFreload=Zero  ePWNxBOutWay=off  ePWMxLINKCMPA=Not Linked  CMPAUnits=Clock cycles  CMPASource=Input port  CMPAValue_per=32000  CMPAValue_clk=target.PWM_Counter_Period/2+1  enCMPAshadow=Counter equals to zero (CTR=Zero)  ePWMxLINKCMPB=Not Linked  CMPBUnits=Clock cycles  CMPBSource=Specify via dialog  CMPBValue_per=50  CMPBValue_clk=target.PWM_Counter_Period/2+1  enCMPBshadow=Counter equals to zero (CTR=Zero)  ePWMxLINKCMPC=Not Linked  CMPCUnits=Clock cycles  CMPCSource=Specify via dialog  CMPCValue_per=50  CMPCValue_clk=32000  enCMPCshadow=Counter equals to zero (CTR=Zero)  ePWMxLINKCMPD=Not Linked  CMPDUnits=Clock cycles  CMPDSource=Specify via dialog  CMPDValue_per=50  CMPDValue_clk=32000  enCMPDshadow=Counter equals to zero (CTR=Zero)  enableDBePWMxA=on  enableDBePWMxB=on  enhalfcycle=off  DBpolarity=Active high complementary (AHC)  DBedgeDelay=Positive  DBSource_ePWMxA=ePWMxA  DBSource_ePWMxB=ePWMxA  DBPeriodUnits=Clock cycles  DBperiodSource=Specify via dialog  REDperiod=15  FEDperiod=15  REDperiod_sec=0  FEDperiod_sec=0  LoadModeDBRED=Immediate without using shadow  LoadModeDBFED=Immediate without using shadow  adcstartModuleA=off  adcrequestEventA=First event  adcstartEventA=Digital Compare Module A Event 1 start of conversion (DCAEVT1.soc)  adcstartEventA_type2=Digital Compare Module A Event 1 start of conversion (DCAEVT1.soc)  adcstartModuleB=off  adcrequestEventB=First event  adcstartEventB=Counter equals to zero (CTR=Zero)  adcstartEventB_type2=Counter equals to zero (CTR=Zero)  intEn=off  intPrd=First event  intSel=Counter equals to zero (CTR=Zero)  intSel_type2=Counter equals to zero (CTR=Zero)  hrpe=off  enHRPWM=off  HRPWM_LoadMode=Counter equals to period (CTR=PRD)  HRPWM_CTLMode=Duty or Period control mode  HRPWM_EDGMode=Both edge  hrpeb=off  enHRPWMB=off  HRPWM_LoadModeB=Counter equals to zero (CTR=ZERO)  HRPWM_CTLModeB=Duty or Period control mode  HRPWM_EDGModeB=Both edge  enHRDBRED=off  enHRDBFED=off  enSFO=on  enautoconv=on  chopperEnable=off  chopperFrequency=1  chopperFirstwidth=1  chopperDuty=12.5%  tripZonesource=Specify via dialog  tzselOSHT1=off  tzselOSHT2=off  tzselOSHT3=off  tzselOSHDCAEV1=off  tzselOSHDCBEV1=off  tzselCBC1=off  tzselCBC2=off  tzselCBC3=off  tzselCBCDCAEV2=off  tzselCBCDCBEV2=off  tzselOSHT4=off  tzselOSHT5=off  tzselOSHT6=off  tzselCBC4=off  tzselCBC5=off  tzselCBC6=off  enTzOstIntr=off  enTzCbcIntr=off  enTzDCAEVT1Intr=off  enTzDCAEVT2Intr=off  enTzDCBEVT1Intr=off  enTzDCBEVT2Intr=off  ePWMxAforced=No action  ePWMxBforced=No action  DCAEVT1forced=No action  DCBEVT1forced=No action  DCAEVT2forced=No action  DCBEVT2forced=No action  dcah=Trip Zone 1 input (TZ1)  dcal=Trip Zone 2 input (TZ2)  dcbh=Trip Zone 1 input (TZ1)  dcbl=Trip Zone 2 input (TZ2)  dcah_type2=GPTRIP1SEL/(TZ1)  dcal_type2=GPTRIP2SEL/(TZ2)  dcbh_type2=GPTRIP1SEL/(TZ1)  dcbl_type2=GPTRIP2SEL/(TZ2)  gendcaevt1=Event disabled  gendcaevt2=Event disabled  gendcbevt1=Event disabled  gendcbevt2=Event disabled  dcaevt1src=DCAEVT1 with sync  dcaevt2src=DCAEVT2 with sync  dcbevt1src=DCBEVT1 with sync  dcbevt2src=DCBEVT2 with sync  pulsesel=Counter equals to zero (CTR=Zero)  blankinv=off  blankoffset=0  blankwidth=0  evsrcsel=Filtered version of DCAEVT1 (DCAEVT1FILT)  encape=off
  ePWM3 : c2802xlib/ePWM  PwmType=C2000  useModule=ePWM3  ePWMxLINKTBPRD=Not Linked  periodUnits=Clock cycles  timerSource=Specify via dialog  timerPeriod_clk=target.PWM_Counter_Period+1  timerPeriod_sec=64000  tbshadow=Counter equals to zero  countingMode=Up-Down  phaseActiveEnable=Set counter to phase value specified via dialog  phaseDirection=Count up after sync  phaseActive=0  synchronizationEnable=off  dcaevt1Sync=off  dcbevt1Sync=off  synchronizationOption=Disable  perSynchronizationOption=Counter equals to period (CTR=PRD)  clockPrescale=1  HSclockPrescale=1  enswap=off  ePWMxAStatus=on  ePWMxAactionLogic1=Do nothing  ePWMxAactionLogic2=Do nothing  ePWMxAactionLogic3=Clear  ePWMxAactionLogic4=Set  ePWMxAactionLogic5=Do nothing  ePWMxAactionLogic6=Do nothing  ePWMxACSFenable=off  ePWMxACSFvalue=Forcing disable  ePWMxASFreload=Zero  ePWMxBStatus=off  ePWMxBactionLogic1=Do nothing  ePWMxBactionLogic2=Set  ePWMxBactionLogic3=Do nothing  ePWMxBactionLogic4=Do nothing  ePWMxBactionLogic5=Clear  ePWMxBactionLogic6=Do nothing  ePWMxBCSFenable=off  ePWMxBCSFvalue=Forcing disable  ePWMxBSFreload=Zero  ePWNxBOutWay=off  ePWMxLINKCMPA=Not Linked  CMPAUnits=Clock cycles  CMPASource=Input port  CMPAValue_per=32000  CMPAValue_clk=target.PWM_Counter_Period/2+1  enCMPAshadow=Counter equals to zero (CTR=Zero)  ePWMxLINKCMPB=Not Linked  CMPBUnits=Clock cycles  CMPBSource=Specify via dialog  CMPBValue_per=50  CMPBValue_clk=target.PWM_Counter_Period/2+1  enCMPBshadow=Counter equals to zero (CTR=Zero)  ePWMxLINKCMPC=Not Linked  CMPCUnits=Clock cycles  CMPCSource=Specify via dialog  CMPCValue_per=50  CMPCValue_clk=32000  enCMPCshadow=Counter equals to zero (CTR=Zero)  ePWMxLINKCMPD=Not Linked  CMPDUnits=Clock cycles  CMPDSource=Specify via dialog  CMPDValue_per=50  CMPDValue_clk=32000  enCMPDshadow=Counter equals to zero (CTR=Zero)  enableDBePWMxA=on  enableDBePWMxB=on  enhalfcycle=off  DBpolarity=Active high complementary (AHC)  DBedgeDelay=Positive  DBSource_ePWMxA=ePWMxA  DBSource_ePWMxB=ePWMxA  DBPeriodUnits=Clock cycles  DBperiodSource=Specify via dialog  REDperiod=15  FEDperiod=15  REDperiod_sec=0  FEDperiod_sec=0  LoadModeDBRED=Immediate without using shadow  LoadModeDBFED=Immediate without using shadow  adcstartModuleA=off  adcrequestEventA=First event  adcstartEventA=Digital Compare Module A Event 1 start of conversion (DCAEVT1.soc)  adcstartEventA_type2=Digital Compare Module A Event 1 start of conversion (DCAEVT1.soc)  adcstartModuleB=off  adcrequestEventB=First event  adcstartEventB=Counter equals to zero (CTR=Zero)  adcstartEventB_type2=Counter equals to zero (CTR=Zero)  intEn=off  intPrd=First event  intSel=Counter equals to zero (CTR=Zero)  intSel_type2=Counter equals to zero (CTR=Zero)  hrpe=off  enHRPWM=off  HRPWM_LoadMode=Counter equals to period (CTR=PRD)  HRPWM_CTLMode=Duty or Period control mode  HRPWM_EDGMode=Both edge  hrpeb=off  enHRPWMB=off  HRPWM_LoadModeB=Counter equals to zero (CTR=ZERO)  HRPWM_CTLModeB=Duty or Period control mode  HRPWM_EDGModeB=Both edge  enHRDBRED=off  enHRDBFED=off  enSFO=on  enautoconv=on  chopperEnable=off  chopperFrequency=1  chopperFirstwidth=1  chopperDuty=12.5%  tripZonesource=Specify via dialog  tzselOSHT1=off  tzselOSHT2=off  tzselOSHT3=off  tzselOSHDCAEV1=off  tzselOSHDCBEV1=off  tzselCBC1=off  tzselCBC2=off  tzselCBC3=off  tzselCBCDCAEV2=off  tzselCBCDCBEV2=off  tzselOSHT4=off  tzselOSHT5=off  tzselOSHT6=off  tzselCBC4=off  tzselCBC5=off  tzselCBC6=off  enTzOstIntr=off  enTzCbcIntr=off  enTzDCAEVT1Intr=off  enTzDCAEVT2Intr=off  enTzDCBEVT1Intr=off  enTzDCBEVT2Intr=off  ePWMxAforced=No action  ePWMxBforced=No action  DCAEVT1forced=No action  DCBEVT1forced=No action  DCAEVT2forced=No action  DCBEVT2forced=No action  dcah=Trip Zone 1 input (TZ1)  dcal=Trip Zone 2 input (TZ2)  dcbh=Trip Zone 1 input (TZ1)  dcbl=Trip Zone 2 input (TZ2)  dcah_type2=GPTRIP1SEL/(TZ1)  dcal_type2=GPTRIP2SEL/(TZ2)  dcbh_type2=GPTRIP1SEL/(TZ1)  dcbl_type2=GPTRIP2SEL/(TZ2)  gendcaevt1=Event disabled  gendcaevt2=Event disabled  gendcbevt1=Event disabled  gendcbevt2=Event disabled  dcaevt1src=DCAEVT1 with sync  dcaevt2src=DCAEVT2 with sync  dcbevt1src=DCBEVT1 with sync  dcbevt2src=DCBEVT2 with sync  pulsesel=Counter equals to zero (CTR=Zero)  blankinv=off  blankoffset=0  blankwidth=0  evsrcsel=Filtered version of DCAEVT1 (DCAEVT1FILT)  encape=off
  stop : Constant  Value=0  OutDataTypeStr=uint16
  sim_duty : Outport  VectorParamsAs1DForOutWhenUnconnected=off
  wires:
  Demux1/3 -> ePWM3/1  "PWM_C"
  Scale_to_PWM_Counter_PRD/1 -> Switch1/1
  Mux2/1 -> Switch1/3
  stop/1 -> Mux2/3, Mux2/2, Mux2/1
  Demux/4 -> Switch1/2  "PWM_Enable"
  Inverter Signals/1 -> Demux/1
  Demux1/2 -> ePWM2/1  "PWM_B"
  Switch1/1 -> Demux1/1
  Demux1/1 -> ePWM1/1  "PWM_A"
  Mux/1 -> Scale_to_PWM_Counter_PRD/1  "PWM Duty Cycles"
  Ground/1 -> Mux1/1
  Ground1/1 -> Mux1/3
  Ground2/1 -> Mux1/2
  Mux1/1 -> sim_duty/1
  Demux/1 -> Mux/1
  Demux/2 -> Mux/2
  Demux/3 -> Mux/3
  INV Enable/1 -> Digital Output2/1

== system mcb_pmsm_foc_hall_hvkit_f28069m/Embedded Processor/Inverter Driver Peripherals/Inverter (Simulation) ==
  Inverter Signals : Inport
  Data Type Duplicate : DataTypeDuplicate
  Demux : Demux
  Mux : Mux  Inputs=3
  Mux2 : Mux  Inputs=3
  Switch1 : Switch  Threshold=0.5  RndMeth=Simplest
  stop : Constant  Value=0  OutDataTypeStr=Inherit: Inherit via back propagation
  sim_duty : Outport  VectorParamsAs1DForOutWhenUnconnected=off
  wires:
  stop/1 -> Data Type Duplicate/2, Mux2/1, Mux2/3, Mux2/2
  Mux2/1 -> Switch1/3
  Switch1/1 -> sim_duty/1
  Inverter Signals/1 -> Demux/1
  Demux/4 -> Switch1/2  "PWM Enable"
  Mux/1 -> Data Type Duplicate/1, Switch1/1  "PWM Duty Cycles"
  Demux/1 -> Mux/1
  Demux/2 -> Mux/2
  Demux/3 -> Mux/3

== system mcb_pmsm_foc_hall_hvkit_f28069m/Embedded Processor/Sensor Driver Blocks/Sensor Driver Blocks (codegen) ==
  Sim_fb : Inport
  Ground : Ground
  IA Measurement : c2802xlib/ADC  blkParamProc=C2000  ADCModule=1  samplingMode=Single sample mode  ADCResolution=12-bit (Single-ended input)  useSOC1=SOC0  useSOC2=SOC0_SOC1  SOCAcquisitionWindow=7  SOCTriggerSource=ePWM1_ADCSOCA  SOCInterruptTrigger=No ADCINT  Ts=-1  dType=uint16  postInterrupt=off  interruptSel=ADCINT1  ADCINTContinuous=on  endma=off  chdma=1  conv1=ADCINB3  conv2=ADCINA1 and ADCINB1  conv1_Type4=ADCIN0  conv2_Type4=ADCIN0 and ADCIN1
  IB Measurement : c2802xlib/ADC  blkParamProc=C2000  ADCModule=1  samplingMode=Single sample mode  ADCResolution=12-bit (Single-ended input)  useSOC1=SOC1  useSOC2=SOC0_SOC1  SOCAcquisitionWindow=7  SOCTriggerSource=ePWM1_ADCSOCA  SOCInterruptTrigger=No ADCINT  Ts=-1  dType=uint16  postInterrupt=on  interruptSel=ADCINT1  ADCINTContinuous=on  endma=off  chdma=1  conv1=ADCINB5  conv2=ADCINA1 and ADCINB1  conv1_Type4=ADCIN0  conv2_Type4=ADCIN0 and ADCIN1
  Mux : Mux  Inputs=2
  Terminator : Terminator
  Iab_Meas_ADC : Outport
  Pos_sim : Outport  Port=2
  wires:
  Mux/1 -> Iab_Meas_ADC/1
  Sim_fb/1 -> Terminator/1
  Ground/1 -> Pos_sim/1
  IA Measurement/1 -> Mux/1
  IB Measurement/1 -> Mux/2

== system mcb_pmsm_foc_hall_hvkit_f28069m/Embedded Processor/Sensor Driver Blocks/Sensor Driver Blocks (sim) ==
  Sim_fb : Inport
  Bus Selector : BusSelector  OutputSignals=Iab_sim,pos_sim
  Iab_Meas_ADC : Outport
  Pos_sim : Outport  Port=2
  wires:
  Sim_fb/1 -> Bus Selector/1
  Bus Selector/1 -> Iab_Meas_ADC/1  "<Iab_sim>"
  Bus Selector/2 -> Pos_sim/1  "<pos_sim>"

== system mcb_pmsm_foc_hall_hvkit_f28069m/Inverter and Motor - Plant Model/Plant Model/Codegeneration ==
  Duty_Cycles : Inport
  Ground : Ground
  Ground1 : Ground
  Terminator : Terminator
  Iab_sim : Outport  VectorParamsAs1DForOutWhenUnconnected=off
  pos_Sim : Outport  Port=2  VectorParamsAs1DForOutWhenUnconnected=off
  wires:
  Duty_Cycles/1 -> Terminator/1
  Ground/1 -> Iab_sim/1
  Ground1/1 -> pos_Sim/1

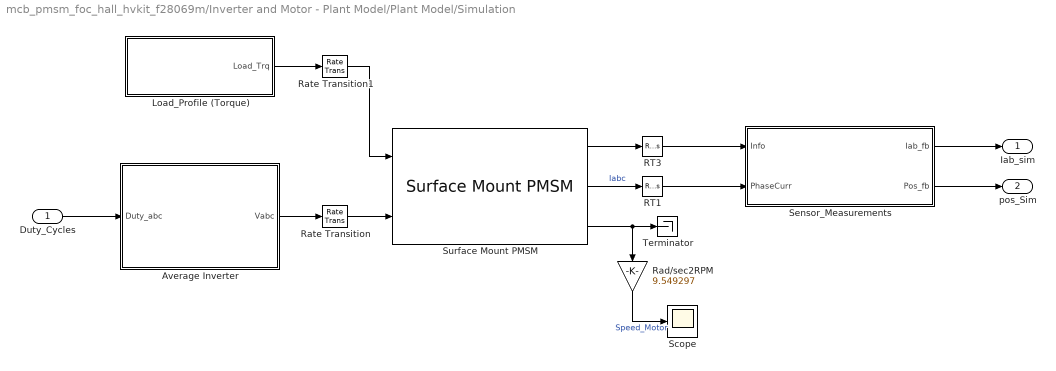
== system mcb_pmsm_foc_hall_hvkit_f28069m/Inverter and Motor - Plant Model/Plant Model/Simulation ==
  Duty_Cycles : Inport
  Average Inverter : Subsystem
  Load_Profile (Torque) : Subsystem
  RT1 : RateTransition  Deterministic=off  OutPortSampleTime=Ts_simulink
  RT3 : RateTransition  Deterministic=off  OutPortSampleTime=Ts_simulink
  Rad/sec2RPM : Gain  Gain=9.549297
  Rate Transition : RateTransition  Integrity=off  OutPortSampleTime=Ts_motor
  Rate Transition1 : RateTransition  Integrity=off  OutPortSampleTime=Ts_motor
  Scope : Scope
  Sensor_Measurements : Subsystem
  Surface Mount PMSM : autolibpmsmexterior/Surface Mount PMSM  port_config=Torque  sim_type=Discrete  Ts=Ts_motor  FilePath=surfacepmsm_motordata.m  P=pmsm.p  Rs=pmsm.Rs  Ldq_=pmsm.Ld  KConstText=Permanent flux linkage constant (lambda_pm):  lambda_pm=pmsm.FluxPM  Ke=159.9771  Kt=1.323  mechanical=[pmsm.J, pmsm.B, 0]  idq0=[0 0]  theta_init=0  omega_init=0  KConst=pmsm.FluxPM  lambda_pm_calc=pmsm.FluxPM  RefBlkName='autolibpmsmexterior/Surface Mount PMSM'  aMode=5  Ldq="[0.00105     0.00105]"
      settings: SourceProductBaseCode=PW,DR,MT,UV,VE
  Terminator : Terminator
  Iab_sim : Outport
  pos_Sim : Outport  Port=2
  wires:
  RT1/1 -> Sensor_Measurements/2(PhaseCurr)
  Surface Mount PMSM/2 -> RT1/1  "Iabc"
  RT3/1 -> Sensor_Measurements/1(Info)
  Rate Transition1/1 -> Surface Mount PMSM/1
  Average Inverter/1(Vabc) -> Rate Transition/1
  Rate Transition/1 -> Surface Mount PMSM/2
  Duty_Cycles/1 -> Average Inverter/1(Duty_abc)
  Surface Mount PMSM/3 -> Rad/sec2RPM/1, Terminator/1
  Surface Mount PMSM/1 -> RT3/1
  Load_Profile (Torque)/1(Load_Trq) -> Rate Transition1/1
  Rad/sec2RPM/1 -> Scope/1  "Speed_Motor"
  Sensor_Measurements/1(Iab_fb) -> Iab_sim/1
  Sensor_Measurements/2(Pos_fb) -> pos_Sim/1
